simulink model "hw10_flyback_wfilter"  (R2017b)
settings: Solver=ode23tb  StartTime=0.0  StopTime=10e-3  RelTol=1e-4  EnableMultiTasking=on
values from neighbouring files (symbols this model uses):
  C = 100e-6    (= 0.0001)    [flyback_filter.m]    (also in hw10_flyback_filter.m)
  Cb = n*Cf    [flyback_filter.m]    (also in hw10_flyback_filter.m = nf*Cf)
  Cf = 47e-6 * 3    (= 0.000141)    [flyback_filter.m]    (also in hw10_flyback_filter.m)
  D = 0.3    [flyback_filter.m]    (also in hw10_flyback_filter.m)
  L = 250e-6    (= 0.00025)    [flyback_filter.m]    (also in hw10_flyback_filter.m)
  Lf = ((1/(fo*2*pi))^2)/Cf    [flyback_filter.m]    (also in hw10_flyback_filter.m = 1/(ff^2)/4/pi/pi/Cf)
  n = (-b + sqrt(b^2 - 4*a*c))/(2*a)    [flyback_filter.m]    (also in hw10_flyback_filter.m = 0.5)
  R = 5    [flyback_filter.m]    (also in hw10_flyback_filter.m)
  Rf = Rof*sqrt( ( (2+n) * (4+3*n) ) / ( (2*n^2) * (4+n) ) )    [flyback_filter.m]    (also in hw10_flyback_filter.m = Rof*sqrt( (2+nf)*(4+3*nf)/(2*nf^2*(4+nf)) ))
  Ts = 1/fsw    (= 5e-06)    [flyback_filter.m]    (also in hw10_flyback_filter.m)
  Vg = 48    [flyback_filter.m]    (also in hw10_flyback_filter.m)
undefined symbols (not defined in the file or in its folder): Cout
libraries: powerlib x17, powerlib_meascontrol x1
settings Model: Creator=jvr2131  LastModifiedBy=jvr2131
settings DataIOCC: LimitDataPoints=on  SaveFormat=Array
settings OptimizationCC: LifeSpan=inf
settings DebuggingCC: UnderspecifiedInitializationDetection=Classic  MergeDetectMultiDrivingBlocksExec=none  SolverPrmCheckMsg=warning  UnconnectedInputMsg=none  UnconnectedOutputMsg=none  UnconnectedLineMsg=none  StateNameClashWarn=warning  SFUnexpectedBacktrackingDiag=warning  SFNoUnconditionalDefaultTransitionDiag=warning  SFExecutionAtInitializationDiag=none
settings HardwareCC: ProdBitPerPointer=32  ProdBitPerSizeT=32  ProdBitPerPtrDiffT=32  ProdLargestAtomicFloat=None  ProdIntDivRoundTo=Undefined  ProdEndianess=Unspecified  ProdWordSize=32  ProdHWDeviceType=32-bit Generic
settings ModelReferenceCC: PropagateSignalLabelsOutOfModel=off
settings CodeAppCC: StateflowObjectComments=on
settings GRTTargetCC: TargetLangStandard=C89/C90 (ANSI)  GeneratePreprocessorConditionals=Disable all
settings ConfigComp: CovMetricSettings=dw  CovHtmlReporting=on  CovSaveCumulativeToWorkspaceVar=on  CovSaveSingleToWorkspaceVar=on  CovExternalEMLEnable=off
settings SimscapeCC: SimscapeNormalizeSystem=off

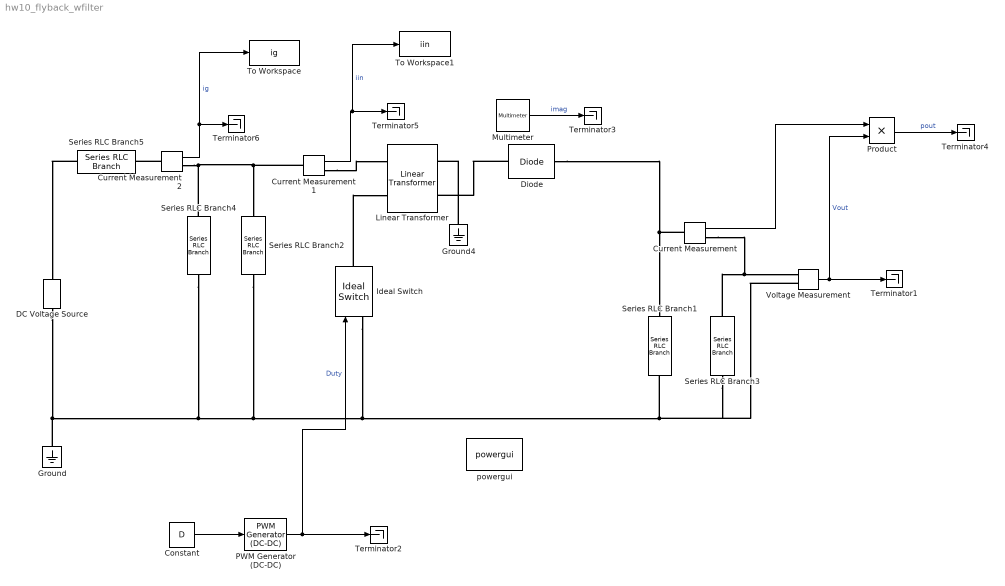
== system hw10_flyback_wfilter ==
  Constant : Constant  Value=D
  Current Measurement : powerlib/Measurements/Current Measurement  PhasorSimulation=off  OutputType=Complex  PSBequivalent=0
  Current Measurement1 : powerlib/Measurements/Current Measurement  PhasorSimulation=off  OutputType=Complex  PSBequivalent=0
  Current Measurement2 : powerlib/Measurements/Current Measurement  PhasorSimulation=off  OutputType=Complex  PSBequivalent=0
  DC Voltage Source : powerlib/Electrical Sources/DC Voltage Source  Amplitude=Vg  Measurements=None
  Diode : powerlib/Power Electronics/Diode  Ron=.0001  Lon=0  Vf=0  IC=0  UseSnubber=off  Rs=500  Cs=0  Measurements=off
  Ground : powerlib/Elements/Ground  LConnTagsString=a
  Ground4 : powerlib/Elements/Ground  LConnTagsString=a
  Ideal Switch : powerlib/Power Electronics/Ideal Switch  Ron=0.00001  Lon=0  IC=0  Rs=1e5  Cs=inf  Measurements=off
  Linear Transformer : powerlib/Elements/Linear Transformer  UNITS=SI  NominalPower=[ 250e6 60 ]  winding1=[7.35e+05 0 0]  winding2=[n*7.35e+05 0 0]  ThreeWindings=off  winding3=[3.15e+05 0.7938 0.084225]  RmLm=[1.0805e+06 L]  Measurements=All voltages and currents  DataType=on
  Multimeter : powerlib/Measurements/Multimeter  PhasorSimulation=off  OutputType=Complex  sel=6  L=7  Gain=1  yselected={'Imag: Linear Transformer'};  PSBOutputType=1  PSBequivalent=0  AxesSetting=[0,0.1,-100,100]  Display=0  SavedBlockNames=-11
  PWM Generator (DC-DC) : powerlib_meascontrol/Pulse & Signal Generators/PWM Generator (DC-DC)  Fsw=fs  Ts=0
  Product : Product
  Series RLC Branch1 : powerlib/Elements/Series RLC Branch  LConnTagsString=__new0  RConnTagsString=__new0  BranchType=C  Resistance=1  Inductance=1e-3  SetiL0=off  InitialCurrent=0  Capacitance=C  Setx0=on  InitialVoltage=V  Measurements=None
  Series RLC Branch2 : powerlib/Elements/Series RLC Branch  LConnTagsString=__new0  RConnTagsString=__new0  BranchType=RC  Resistance=Rf  Inductance=1e-3  SetiL0=off  InitialCurrent=0  Capacitance=Cb  Setx0=off  InitialVoltage=0  Measurements=None
  Series RLC Branch3 : powerlib/Elements/Series RLC Branch  LConnTagsString=__new0  RConnTagsString=__new0  BranchType=R  Resistance=R  Inductance=1e-3  SetiL0=off  InitialCurrent=0  Capacitance=Cout  Setx0=off  InitialVoltage=0  Measurements=None
  Series RLC Branch4 : powerlib/Elements/Series RLC Branch  LConnTagsString=__new0  RConnTagsString=__new0  BranchType=C  Resistance=Rf  Inductance=1e-3  SetiL0=off  InitialCurrent=0  Capacitance=Cf  Setx0=off  InitialVoltage=0  Measurements=None
  Series RLC Branch5 : powerlib/Elements/Series RLC Branch  LConnTagsString=__new0  RConnTagsString=__new0  BranchType=L  Resistance=Rf  Inductance=Lf  SetiL0=off  InitialCurrent=0  Capacitance=Cb  Setx0=off  InitialVoltage=0  Measurements=None
  Terminator{1..6} (6 alike) : Terminator
  To Workspace : ToWorkspace  VariableName=ig  SampleTime=-1
  To Workspace1 : ToWorkspace  VariableName=iin  SampleTime=-1
  Voltage Measurement : powerlib/Measurements/Voltage Measurement  PhasorSimulation=off  OutputType=Complex  PSBequivalent=0
  powergui : powerlib/powergui  Priority=1  SimulationMode=Discrete  SampleTime=Ts/1000  frequency=60  Iterations=50  frequencyindice=0  Pbase=100e6  ErrMax=1e-4  UnitsV=kV  UnitsW=MW  buscounter=0  FunctionMessages=off  echomessages=off  EnableUseOfTLC=off  CurrentSourceSwitches=off  DisableSnubberDevices=off  DisableRonSwitches=off  DisableVfSwitches=off  DisplayEquations=off  SolverType=Tustin  Interpol=off  ExternalGateDelay=off  methode=off  Ts=0  x0status=blocks  SPID=off  SwTol=0  HookPort=off  RestoreLinks=warning  ResistiveCurrentMeasurement=off  Frange=[0:2:500]  Ylog=off  Xlog=on  ShowGrid=off  save=off  variable=ZData  structure=0  ZoomFFT=off  StartTime=0.0  cycles=1  DisplayStyle=1  fundamental=60  FreqAxis=off  MaxFrequency=1000  frequencyindicesteady=1  RmsSteady=1  display=off
  wires:
  Constant/1 -> PWM Generator (DC-DC)/1
  Voltage Measurement/1 -> Product/2, Terminator1/1  "Vout"
  PWM Generator (DC-DC)/1 -> Ideal Switch/1, Terminator2/1  "Duty"
  Multimeter/1 -> Terminator3/1  "imag"
  Current Measurement/1 -> Product/1
  Product/1 -> Terminator4/1  "pout"
  Current Measurement1/1 -> To Workspace1/1, Terminator5/1  "iin"
  Current Measurement2/1 -> To Workspace/1, Terminator6/1  "ig"
  connections:
  Diode/RConn1 -- Current Measurement/LConn1 -- Series RLC Branch1/LConn1
  DC Voltage Source/LConn1 -- Series RLC Branch4/RConn1 -- Series RLC Branch2/RConn1 -- Ideal Switch/LConn1 -- Series RLC Branch3/LConn1 -- Voltage Measurement/LConn2 -- Series RLC Branch1/RConn1 -- Ground/LConn1
  Diode/LConn1 -- Linear Transformer/RConn2
  Ground4/LConn1 -- Linear Transformer/RConn1
  Series RLC Branch3/RConn1 -- Current Measurement/RConn1 -- Voltage Measurement/LConn1
  Ideal Switch/RConn1 -- Linear Transformer/LConn2
  Series RLC Branch4/LConn1 -- Current Measurement2/RConn1 -- Current Measurement1/LConn1 -- Series RLC Branch2/LConn1
  Current Measurement1/RConn1 -- Linear Transformer/LConn1
  Current Measurement2/LConn1 -- Series RLC Branch5/LConn1
  Series RLC Branch5/RConn1 -- DC Voltage Source/RConn1
